simulink model "ADRC_3RD_TEST"  (Simulink 7.6)
settings: Solver=ode45  StartTime=0.0  StopTime=100  RelTol=1e-3
libraries: ADRC x1
settings Model: Creator=Administrator  LastModifiedBy=Administrator
settings DebuggingCC: AlgebraicLoopMsg=none  ArtificialAlgebraicLoopMsg=none  SolverPrmCheckMsg=none  UnknownTsInhSupMsg=none

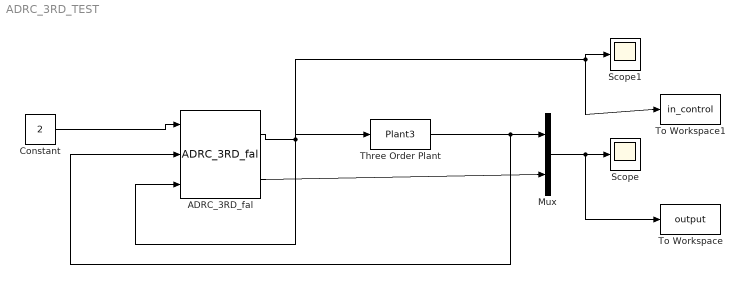
== system ADRC_3RD_TEST ==
  ADRC_3RD_fal : ADRC/ADRC/ADRC_3rd/ADRC_3RD_fal  SystemSampleTime=-1  h=0.01  TD=[0.5,0.01]  ESO=[100,60,100,400,0.0001]  NLSEF=[80,20,5,0.01]  b0=1
  Constant : Constant  Value=2
  Mux : Mux  Inputs=2
  Scope : Scope
      settings: TimeRange=20  YMin=1.35  YMax=2.5  DataFormat=Array
  Scope1 : Scope
      settings: TimeRange=50  YMin=1.8  YMax=2.1  DataFormat=Array
  Three Order Plant : S-Function  FunctionName=Plant3  EnableBusSupport=off
  To Workspace : ToWorkspace  VariableName=output  SampleTime=1  SaveFormat=Array
  To Workspace1 : ToWorkspace  VariableName=in_control  SampleTime=1  SaveFormat=Array
  wires:
  ADRC_3RD_fal/1 -> Scope1/1, To Workspace1/1, Three Order Plant/1, ADRC_3RD_fal/3
  Three Order Plant/1 -> Mux/1, ADRC_3RD_fal/2
  ADRC_3RD_fal/2 -> Mux/2
  Mux/1 -> To Workspace/1, Scope/1
  Constant/1 -> ADRC_3RD_fal/1
